simulink model "modelSimulink"  (R2020b)
settings: Solver=VariableStepAuto  StartTime=0.0  StopTime=100  RelTol=1e-3
settings Model: Creator=Sebastian  LastModifiedBy=Sebastian

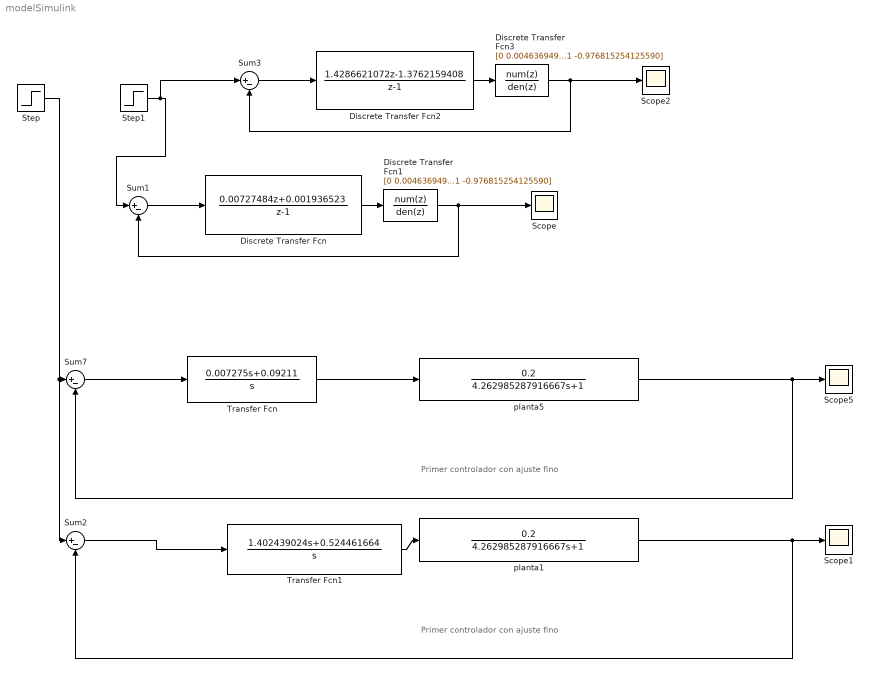
== system modelSimulink ==
  note: Primer controlador con ajuste fino
  note: Primer controlador con ajuste fino
  Discrete Transfer Fcn : DiscreteTransferFcn  Numerator=[0.00727484 0.001936523]  Denominator=[1 -1]  SampleTime=0.1
  Discrete Transfer Fcn1 : DiscreteTransferFcn  Numerator=[0 0.004636949174882]  Denominator=[1 -0.976815254125590]  SampleTime=0.1
  Discrete Transfer Fcn2 : DiscreteTransferFcn  Numerator=[1.4286621072 -1.3762159408]  Denominator=[1 -1]  SampleTime=0.1
  Discrete Transfer Fcn3 : DiscreteTransferFcn  Numerator=[0 0.004636949174882]  Denominator=[1 -0.976815254125590]  SampleTime=0.1
  Scope{,1..2,5} (4 alike) : Scope
  Step : Step  Time=0  SampleTime=0
  Step1 : Step  SampleTime=0.1
  Sum{1..3,7} (4 alike) : Sum  Inputs=|+-
  Transfer Fcn : TransferFcn  Numerator=[0.007275 0.09211]  Denominator=[1 0]
  Transfer Fcn1 : TransferFcn  Numerator=[1.402439024 0.524461664]  Denominator=[1 0]
  planta1 : TransferFcn  Numerator=[0.2]  Denominator=[4.262985287916667 1]
  planta5 : TransferFcn  Numerator=[0.2]  Denominator=[4.262985287916667 1]
  wires:
  Step/1 -> Sum2/1, Sum7/1
  planta5/1 -> Sum7/2, Scope5/1
  Sum1/1 -> Discrete Transfer Fcn/1
  Discrete Transfer Fcn/1 -> Discrete Transfer Fcn1/1
  Step1/1 -> Sum3/1, Sum1/1
  Discrete Transfer Fcn1/1 -> Scope/1, Sum1/2
  Sum7/1 -> Transfer Fcn/1
  Transfer Fcn/1 -> planta5/1
  Transfer Fcn1/1 -> planta1/1
  Sum2/1 -> Transfer Fcn1/1
  planta1/1 -> Sum2/2, Scope1/1
  Discrete Transfer Fcn2/1 -> Discrete Transfer Fcn3/1
  Sum3/1 -> Discrete Transfer Fcn2/1
  Discrete Transfer Fcn3/1 -> Scope2/1, Sum3/2
